simulink model "deadzone_without_offset"  (R2016b)
settings: Solver=VariableStepAuto  StartTime=0.0  StopTime=4  RelTol=1e-3
settings Model: Creator=pong0923  LastModifiedBy=pong0923

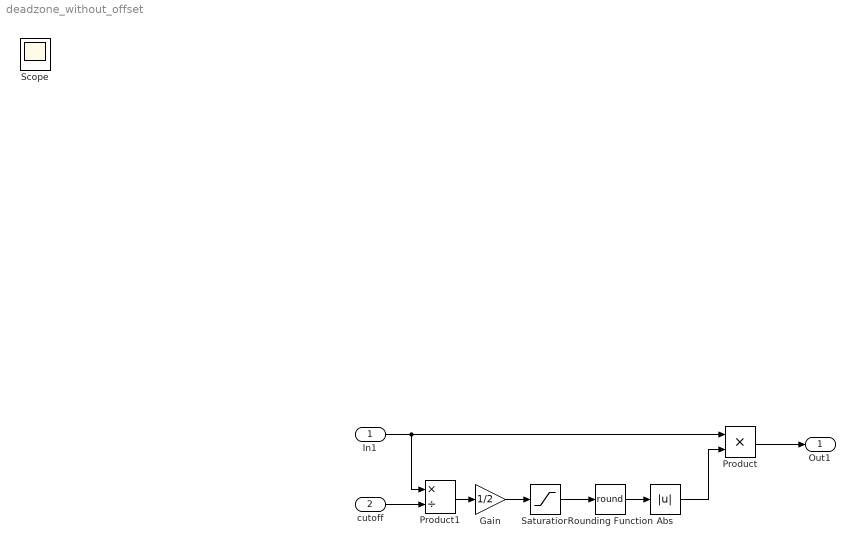
== system deadzone_without_offset ==
  In1 : Inport
  cutoff : Inport  Port=2
  Abs : Abs
  Gain : Gain  Gain=1/2
  Product : Product
  Product1 : Product  Inputs=*/
  Rounding Function : Rounding  Operator=round
  Saturation : Saturate
  Out1 : Outport
  Scope : Scope
  wires:
  Saturation/1 -> Rounding Function/1
  Product/1 -> Out1/1
  Rounding Function/1 -> Abs/1
  Gain/1 -> Saturation/1
  Abs/1 -> Product/2
  Product1/1 -> Gain/1
  cutoff/1 -> Product1/2
  In1/1 -> Product1/1, Product/1
